simulink model "m02_PMSM_HDL"  (R2023b)
settings: Solver=FixedStepDiscrete  StartTime=0.0  StopTime=0.6  RelTol=1e-3  AbsTol=1e-3
PreLoadFcn:
  | control_data;
  | pmsm_data;
  | 
  | avgFactor = 1;
undefined symbols (not defined in the file): ee_sli_rtmsupport, f1478573793584, f1859323186544, fsw, gcbh, J, Ld, Lq, N, PM, Pmax, Tmax, Ts, Tsc
libraries: hdlssclib x24, simulink x8, SimscapeFPGAHIL_lib x6, fpga_utils_lib x5, hdlsllib x4, eeTransforms x2, eePwmGeneratorTwoLevel x1, eePmsmCurrentController x1, eePmsmCurrentReferenceGen x1, eeVelocityController x1
(part 3 of 3)

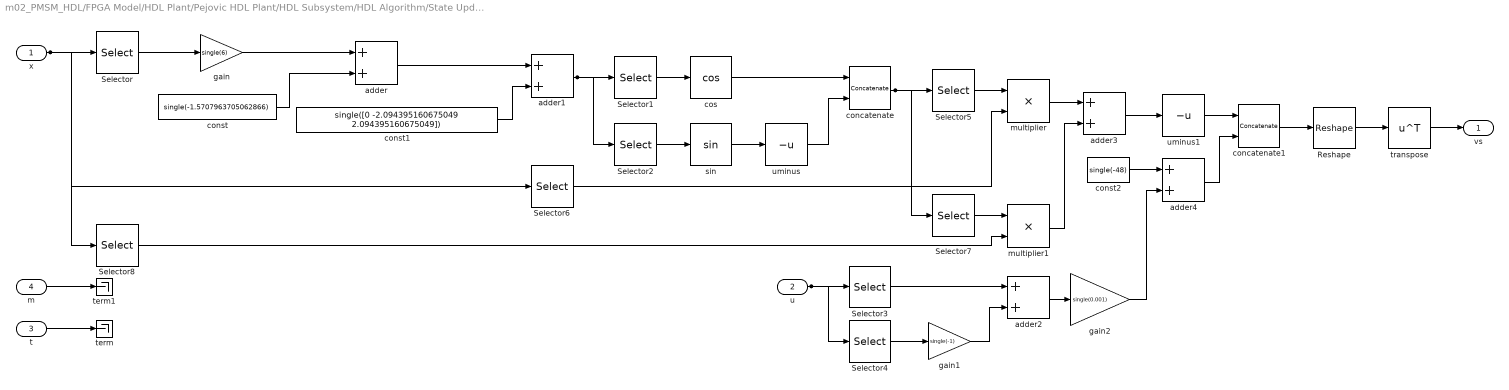
== system m02_PMSM_HDL/FPGA Model/HDL Plant/Pejovic HDL Plant/HDL Subsystem/HDL Algorithm/State Update/Algebraic Clump4/extClump3_F ==
  x : Inport  OutDataTypeStr=single  PortDimensions=[5 1]  SampleTime=2.5e-06
  u : Inport  Port=2  OutDataTypeStr=single  PortDimensions=[2 1]  SampleTime=2.5e-06
  t : Inport  Port=3  OutDataTypeStr=single  SampleTime=2.5e-06
  m : Inport  Port=4  OutDataTypeStr=int32  SampleTime=2.5e-06
  Reshape : Reshape  OutputDimensionality=Column vector (2-D)
  Selector : Selector  SampleTime=2.5e-06  IndexOptions=Index vector (dialog)  Indices=double(3)  OutputSizes=double(0)
  Selector{1..3,5} (4 alike) : Selector  SampleTime=2.5e-06  IndexOptions=Index vector (dialog)  Indices=double(1)  OutputSizes=double(0)
  Selector4 : Selector  SampleTime=2.5e-06  IndexOptions=Index vector (dialog)  Indices=double(2)  OutputSizes=double(0)
  Selector6 : Selector  SampleTime=2.5e-06  IndexOptions=Index vector (dialog)  Indices=double(4)  OutputSizes=double(0)
  Selector7 : Selector  SampleTime=2.5e-06  IndexOptions=Index vector (dialog)  Indices=double(2)  OutputSizes=double(0)
  Selector8 : Selector  SampleTime=2.5e-06  IndexOptions=Index vector (dialog)  Indices=double(5)  OutputSizes=double(0)
  adder{,1..4} (5 alike) : Sum  OutDataTypeStr=single  AccumDataTypeStr=single  SampleTime=2.5e-06
  concatenate : Concatenate  Mode=Multidimensional array  ConcatenateDimension=2
  concatenate1 : Concatenate  Mode=Multidimensional array
  const : Constant  Value=single(-1.5707963705062866)  VectorParams1D=off  OutDataTypeStr=single  SampleTime=2.5e-06
  const1 : Constant  Value=single([0 -2.094395160675049 2.094395160675049])  VectorParams1D=off  OutDataTypeStr=single  SampleTime=2.5e-06
  const2 : Constant  Value=single(-48)  VectorParams1D=off  OutDataTypeStr=single  SampleTime=2.5e-06
  cos : Trigonometry  Operator=cos  SampleTime=2.5e-06
  gain : Gain  Gain=single(6)  OutDataTypeStr=single  SampleTime=2.5e-06
  gain1 : Gain  Gain=single(-1)  OutDataTypeStr=single  SampleTime=2.5e-06
  gain2 : Gain  Gain=single(0.001)  OutDataTypeStr=single  SampleTime=2.5e-06
  multiplier : Product  Inputs=**  OutDataTypeStr=single  SampleTime=2.5e-06
  multiplier1 : Product  Inputs=**  OutDataTypeStr=single  SampleTime=2.5e-06
  sin : Trigonometry  SampleTime=2.5e-06
  term : Terminator
  term1 : Terminator
  transpose : Math  Operator=transpose
  uminus : UnaryMinus  SampleTime=2.5e-06
  uminus1 : UnaryMinus  SampleTime=2.5e-06
  vs : Outport  OutDataTypeStr=single  PortDimensions=[1 2]  SampleTime=2.5e-06
  wires:
  u/1 -> Selector4/1, Selector3/1
  x/1 -> Selector6/1, Selector8/1, Selector/1
  m/1 -> term1/1
  t/1 -> term/1
  Reshape/1 -> transpose/1
  Selector/1 -> gain/1
  Selector7/1 -> multiplier1/1
  Selector8/1 -> multiplier1/2
  cos/1 -> concatenate/1
  gain/1 -> adder/1
  const2/1 -> adder4/1
  const1/1 -> adder1/2
  const/1 -> adder/2
  adder/1 -> adder1/1
  adder2/1 -> gain2/1
  adder1/1 -> Selector2/1, Selector1/1
  Selector5/1 -> multiplier/1
  Selector6/1 -> multiplier/2
  Selector2/1 -> sin/1
  Selector1/1 -> cos/1
  multiplier1/1 -> adder3/2
  sin/1 -> uminus/1
  transpose/1 -> vs/1
  uminus/1 -> concatenate/2
  concatenate1/1 -> Reshape/1
  concatenate/1 -> Selector7/1, Selector5/1
  Selector4/1 -> gain1/1
  Selector3/1 -> adder2/1
  gain2/1 -> adder4/2
  gain1/1 -> adder2/2
  multiplier/1 -> adder3/1
  adder3/1 -> uminus1/1
  uminus1/1 -> concatenate1/1
  adder4/1 -> concatenate1/2

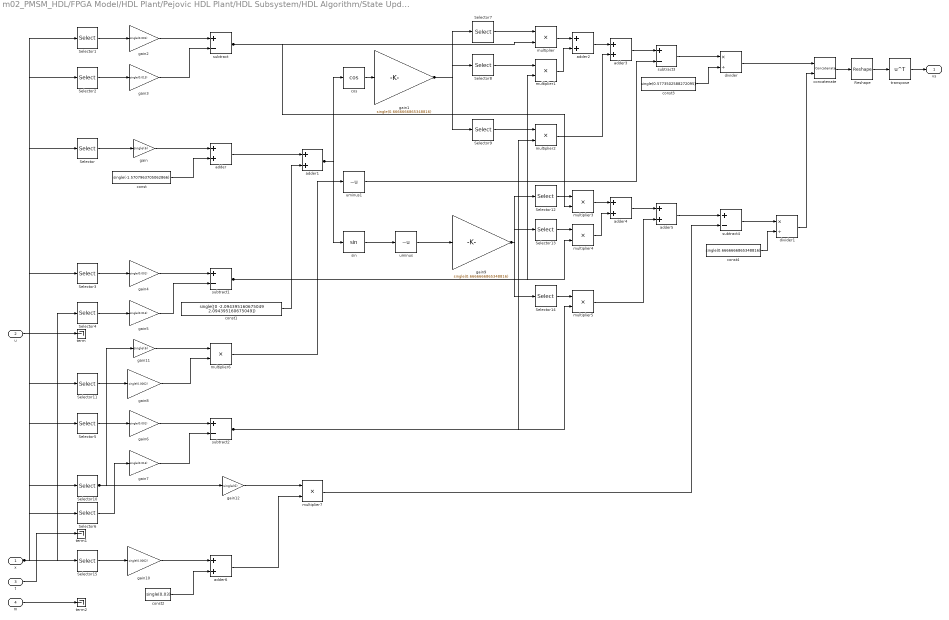
== system m02_PMSM_HDL/FPGA Model/HDL Plant/Pejovic HDL Plant/HDL Subsystem/HDL Algorithm/State Update/Differential Clump/diffClump_F ==
  x : Inport  OutDataTypeStr=single  PortDimensions=[12 1]  SampleTime=2.5e-06
  u : Inport  Port=2  OutDataTypeStr=single  PortDimensions=[6 1]  SampleTime=2.5e-06
  t : Inport  Port=3  OutDataTypeStr=single  SampleTime=2.5e-06
  m : Inport  Port=4  OutDataTypeStr=int32  SampleTime=2.5e-06
  Reshape : Reshape  OutputDimensionality=Column vector (2-D)
  Selector : Selector  SampleTime=2.5e-06  IndexOptions=Index vector (dialog)  Indices=double(10)  OutputSizes=double(0)
  Selector1 : Selector  SampleTime=2.5e-06  IndexOptions=Index vector (dialog)  Indices=double(1)  OutputSizes=double(0)
  Selector10 : Selector  SampleTime=2.5e-06  IndexOptions=Index vector (dialog)  Indices=double(7)  OutputSizes=double(0)
  Selector11 : Selector  SampleTime=2.5e-06  IndexOptions=Index vector (dialog)  Indices=double(12)  OutputSizes=double(0)
  Selector12 : Selector  SampleTime=2.5e-06  IndexOptions=Index vector (dialog)  Indices=double(1)  OutputSizes=double(0)
  Selector13 : Selector  SampleTime=2.5e-06  IndexOptions=Index vector (dialog)  Indices=double(2)  OutputSizes=double(0)
  Selector14 : Selector  SampleTime=2.5e-06  IndexOptions=Index vector (dialog)  Indices=double(3)  OutputSizes=double(0)
  Selector15 : Selector  SampleTime=2.5e-06  IndexOptions=Index vector (dialog)  Indices=double(11)  OutputSizes=double(0)
  Selector2 : Selector  SampleTime=2.5e-06  IndexOptions=Index vector (dialog)  Indices=double(4)  OutputSizes=double(0)
  Selector3 : Selector  SampleTime=2.5e-06  IndexOptions=Index vector (dialog)  Indices=double(2)  OutputSizes=double(0)
  Selector4 : Selector  SampleTime=2.5e-06  IndexOptions=Index vector (dialog)  Indices=double(5)  OutputSizes=double(0)
  Selector5 : Selector  SampleTime=2.5e-06  IndexOptions=Index vector (dialog)  Indices=double(3)  OutputSizes=double(0)
  Selector6 : Selector  SampleTime=2.5e-06  IndexOptions=Index vector (dialog)  Indices=double(6)  OutputSizes=double(0)
  Selector7 : Selector  SampleTime=2.5e-06  IndexOptions=Index vector (dialog)  Indices=double(1)  OutputSizes=double(0)
  Selector8 : Selector  SampleTime=2.5e-06  IndexOptions=Index vector (dialog)  Indices=double(2)  OutputSizes=double(0)
  Selector9 : Selector  SampleTime=2.5e-06  IndexOptions=Index vector (dialog)  Indices=double(3)  OutputSizes=double(0)
  adder{,1..6} (7 alike) : Sum  OutDataTypeStr=single  AccumDataTypeStr=single  SampleTime=2.5e-06
  concatenate : Concatenate  Mode=Multidimensional array
  const : Constant  Value=single(-1.5707963705062866)  VectorParams1D=off  OutDataTypeStr=single  SampleTime=2.5e-06
  const1 : Constant  Value=single([0 -2.094395160675049 2.094395160675049])  VectorParams1D=off  OutDataTypeStr=single  SampleTime=2.5e-06
  const2 : Constant  Value=single(0.03)  VectorParams1D=off  OutDataTypeStr=single  SampleTime=2.5e-06
  const3 : Constant  Value=single(0.5773502588272095)  VectorParams1D=off  OutDataTypeStr=single  SampleTime=2.5e-06
  const4 : Constant  Value=single(0.6666666865348816)  VectorParams1D=off  OutDataTypeStr=single  SampleTime=2.5e-06
  cos : Trigonometry  Operator=cos  SampleTime=2.5e-06
  divider : Product  Inputs=*/  OutDataTypeStr=single  SampleTime=2.5e-06
  divider1 : Product  Inputs=*/  OutDataTypeStr=single  SampleTime=2.5e-06
  gain : Gain  Gain=single(6)  OutDataTypeStr=single  SampleTime=2.5e-06
  gain1 : Gain  Gain=single(0.6666666865348816)  OutDataTypeStr=single  SampleTime=2.5e-06
  gain10 : Gain  Gain=single(0.0002)  OutDataTypeStr=single  SampleTime=2.5e-06
  gain11 : Gain  Gain=single(6)  OutDataTypeStr=single  SampleTime=2.5e-06
  gain12 : Gain  Gain=single(6)  OutDataTypeStr=single  SampleTime=2.5e-06
  gain2 : Gain  Gain=single(0.001)  OutDataTypeStr=single  SampleTime=2.5e-06
  gain3 : Gain  Gain=single(0.013)  OutDataTypeStr=single  SampleTime=2.5e-06
  gain4 : Gain  Gain=single(0.001)  OutDataTypeStr=single  SampleTime=2.5e-06
  gain5 : Gain  Gain=single(0.013)  OutDataTypeStr=single  SampleTime=2.5e-06
  gain6 : Gain  Gain=single(0.001)  OutDataTypeStr=single  SampleTime=2.5e-06
  gain7 : Gain  Gain=single(0.013)  OutDataTypeStr=single  SampleTime=2.5e-06
  gain8 : Gain  Gain=single(0.0002)  OutDataTypeStr=single  SampleTime=2.5e-06
  gain9 : Gain  Gain=single(0.6666666865348816)  OutDataTypeStr=single  SampleTime=2.5e-06
  multiplier{,1..7} (8 alike) : Product  Inputs=**  OutDataTypeStr=single  SampleTime=2.5e-06
  sin : Trigonometry  SampleTime=2.5e-06
  subtract{,1..4} (5 alike) : Sum  Inputs=+-  OutDataTypeStr=single  AccumDataTypeStr=single  SampleTime=2.5e-06
  term : Terminator
  term1 : Terminator
  term2 : Terminator
  transpose : Math  Operator=transpose
  uminus : UnaryMinus  SampleTime=2.5e-06
  uminus1 : UnaryMinus  SampleTime=2.5e-06
  vs : Outport  OutDataTypeStr=single  PortDimensions=[1 2]  SampleTime=2.5e-06
  wires:
  u/1 -> term/1
  t/1 -> term1/1
  adder5/1 -> subtract4/1
  x/1 -> Selector6/1, Selector3/1, Selector1/1, Selector4/1, Selector15/1, Selector2/1, Selector5/1, Selector/1, Selector11/1, Selector10/1
  m/1 -> term2/1
  Selector1/1 -> gain2/1
  Selector/1 -> gain/1
  Selector2/1 -> gain3/1
  Selector3/1 -> gain4/1
  gain3/1 -> subtract/2
  gain2/1 -> subtract/1
  Selector5/1 -> gain6/1
  Selector4/1 -> gain5/1
  Selector10/1 -> gain12/1, gain11/1
  divider/1 -> concatenate/1
  Selector11/1 -> gain8/1
  adder4/1 -> adder5/1
  Selector7/1 -> multiplier/1
  Selector6/1 -> gain7/1
  Selector14/1 -> multiplier5/1
  Selector15/1 -> gain10/1
  divider1/1 -> concatenate/2
  gain/1 -> adder/1
  const3/1 -> divider/2
  const1/1 -> adder1/2
  const2/1 -> adder6/2
  const/1 -> adder/2
  gain5/1 -> subtract1/2
  gain4/1 -> subtract1/1
  gain12/1 -> multiplier7/1
  gain11/1 -> multiplier6/1
  gain9/1 -> Selector14/1, Selector12/1, Selector13/1
  gain8/1 -> multiplier6/2
  gain7/1 -> subtract2/2
  gain6/1 -> subtract2/1
  gain1/1 -> Selector8/1, Selector7/1, Selector9/1
  gain10/1 -> adder6/1
  sin/1 -> uminus/1
  subtract/1 -> multiplier/2, multiplier3/2
  adder/1 -> adder1/1
  subtract1/1 -> multiplier4/2, multiplier1/2
  multiplier5/1 -> adder5/2
  multiplier6/1 -> uminus1/1
  subtract2/1 -> multiplier5/2, multiplier2/2
  adder6/1 -> multiplier7/2
  adder1/1 -> sin/1, cos/1
  multiplier7/1 -> subtract4/2
  const4/1 -> divider1/2
  cos/1 -> gain1/1
  uminus1/1 -> subtract3/2
  uminus/1 -> gain9/1
  Selector9/1 -> multiplier2/1
  Selector8/1 -> multiplier1/1
  multiplier/1 -> adder2/1
  multiplier2/1 -> adder3/2
  multiplier1/1 -> adder2/2
  Selector13/1 -> multiplier4/1
  Selector12/1 -> multiplier3/1
  adder3/1 -> subtract3/1
  adder2/1 -> adder3/1
  multiplier3/1 -> adder4/1
  multiplier4/1 -> adder4/2
  subtract4/1 -> divider1/1
  subtract3/1 -> divider/1
  concatenate/1 -> Reshape/1
  Reshape/1 -> transpose/1
  transpose/1 -> vs/1

== system m02_PMSM_HDL/FPGA Model/HDL Plant/Standard HDL Plant/HDL Subsystem/HDL Algorithm/State Update/Algebraic Clump1/extClump0_F ==
  x : Inport  OutDataTypeStr=single  PortDimensions=[6 1]  SampleTime=2.5e-06
  u : Inport  Port=2  OutDataTypeStr=single  SampleTime=2.5e-06
  t : Inport  Port=3  OutDataTypeStr=single  SampleTime=2.5e-06
  m : Inport  Port=4  OutDataTypeStr=int32  SampleTime=2.5e-06
  Reshape : Reshape  OutputDimensionality=Column vector (2-D)
  Selector : Selector  IndexOptions=Index vector (dialog)  Indices=double(5)  OutputSizes=double(0)
  Selector1 : Selector  IndexOptions=Index vector (dialog)  Indices=double(6)  OutputSizes=double(0)
  Selector2 : Selector  IndexOptions=Index vector (dialog)  Indices=double(6)  OutputSizes=double(0)
  Selector3 : Selector  IndexOptions=Index vector (dialog)  Indices=double(5)  OutputSizes=double(0)
  adder : Sum  OutDataTypeStr=single  AccumDataTypeStr=single  SampleTime=2.5e-06
  concatenate : Concatenate  NumInputs=4  Mode=Multidimensional array
  const : Constant  Value=single(0.03)  VectorParams1D=off  OutDataTypeStr=single  SampleTime=2.5e-06
  const1 : Constant  Value=single(0)  VectorParams1D=off  OutDataTypeStr=single  SampleTime=2.5e-06
  const2 : Constant  Value=single(0)  VectorParams1D=off  OutDataTypeStr=single  SampleTime=2.5e-06
  const3 : Constant  Value=single(0)  VectorParams1D=off  OutDataTypeStr=single  SampleTime=2.5e-06
  gain : Gain  Gain=single(0.0002)  OutDataTypeStr=single  SampleTime=2.5e-06
  gain1 : Gain  Gain=single(0.0002)  OutDataTypeStr=single  SampleTime=2.5e-06
  gain2 : Gain  Gain=single(9)  OutDataTypeStr=single  SampleTime=2.5e-06
  multiplier : Product  Inputs=**  OutDataTypeStr=single  SampleTime=2.5e-06
  multiplier1 : Product  Inputs=**  OutDataTypeStr=single  SampleTime=2.5e-06
  subtract : Sum  Inputs=+-  OutDataTypeStr=single  AccumDataTypeStr=single  SampleTime=2.5e-06
  term : Terminator
  term1 : Terminator
  term2 : Terminator
  transpose : Math  Operator=transpose
  uminus : UnaryMinus  SampleTime=2.5e-06
  vs : Outport  OutDataTypeStr=single  PortDimensions=[1 4]  SampleTime=2.5e-06
  wires:
  u/1 -> term/1
  x/1 -> Selector3/1, Selector2/1, Selector1/1, Selector/1
  t/1 -> term1/1
  m/1 -> term2/1
  const1/1 -> concatenate/2
  const/1 -> adder/2
  Selector/1 -> gain/1
  Selector1/1 -> gain1/1
  gain/1 -> adder/1
  Selector3/1 -> multiplier1/1
  gain1/1 -> multiplier1/2
  Selector2/1 -> multiplier/1
  adder/1 -> multiplier/2
  multiplier1/1 -> subtract/2
  multiplier/1 -> subtract/1
  transpose/1 -> vs/1
  subtract/1 -> gain2/1
  gain2/1 -> uminus/1
  uminus/1 -> concatenate/1
  const3/1 -> concatenate/4
  const2/1 -> concatenate/3
  concatenate/1 -> Reshape/1
  Reshape/1 -> transpose/1

== system m02_PMSM_HDL/FPGA Model/HDL Plant/Standard HDL Plant/HDL Subsystem/HDL Algorithm/State Update/Algebraic Clump2/Mode Vector To Index ==
  In1 : Inport
  State Mode Vector To Index : hdlssclib/HDL Logic Table  InputTable=[1 0;0 1]  OutputTable=[false;true]
  assertion : Assertion  StopWhenAssertionFail=off
  concat : hdlsllib/Logic and Bit Operations/Bit Concat  numInputs=1
  uncatalogued mode identifier : hdlssclib/HDL Logic Table  InputTable=[1 0;0 1]  OutputTable=[1;1]
  Out1 : Outport  VectorParamsAs1DForOutWhenUnconnected=off
  wires:
  State Mode Vector To Index/1 -> concat/1
  In1/1 -> State Mode Vector To Index/1, uncatalogued mode identifier/1
  uncatalogued mode identifier/1 -> assertion/1
  concat/1 -> Out1/1

== system m02_PMSM_HDL/FPGA Model/HDL Plant/Standard HDL Plant/HDL Subsystem/HDL Algorithm/State Update/Algebraic Clump2/Mode Vector Type Conversion ==
  Mode vec : Inport
  Data Type Conversion : DataTypeConversion  OutDataTypeStr=boolean  RndMeth=Nearest  SaturateOnIntegerOverflow=off
  Out1 : Outport  VectorParamsAs1DForOutWhenUnconnected=off
  wires:
  Mode vec/1 -> Data Type Conversion/1
  Data Type Conversion/1 -> Out1/1

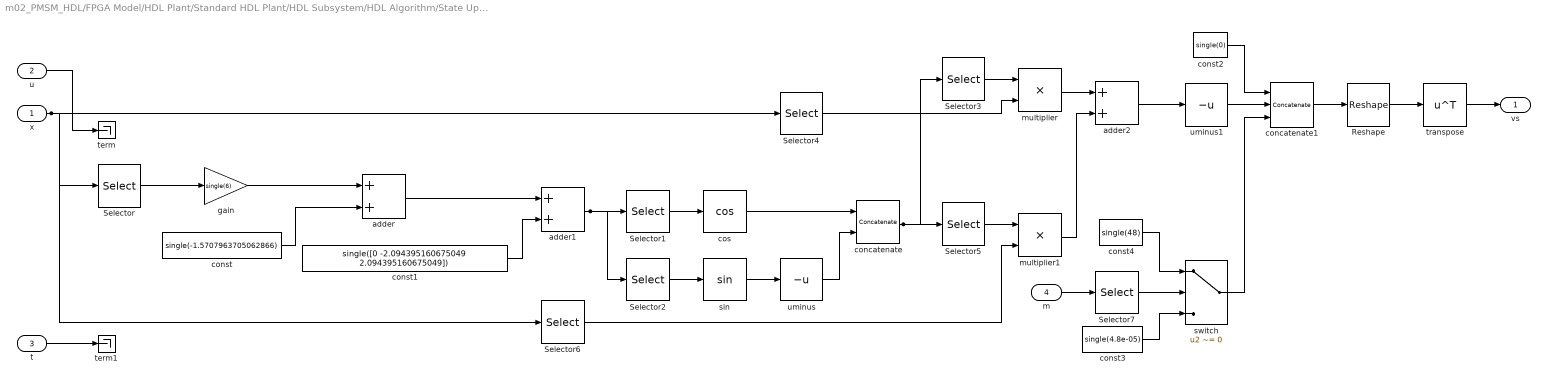
== system m02_PMSM_HDL/FPGA Model/HDL Plant/Standard HDL Plant/HDL Subsystem/HDL Algorithm/State Update/Algebraic Clump2/extClump1_F ==
  x : Inport  OutDataTypeStr=single  PortDimensions=[6 1]  SampleTime=2.5e-06
  u : Inport  Port=2  OutDataTypeStr=single  PortDimensions=[2 1]  SampleTime=2.5e-06
  t : Inport  Port=3  OutDataTypeStr=single  SampleTime=2.5e-06
  m : Inport  Port=4  OutDataTypeStr=int32  PortDimensions=[2 1]  SampleTime=2.5e-06
  Reshape : Reshape  OutputDimensionality=Column vector (2-D)
  Selector : Selector  IndexOptions=Index vector (dialog)  Indices=double(4)  OutputSizes=double(0)
  Selector1 : Selector  IndexOptions=Index vector (dialog)  Indices=double(3)  OutputSizes=double(0)
  Selector2 : Selector  IndexOptions=Index vector (dialog)  Indices=double(3)  OutputSizes=double(0)
  Selector3 : Selector  IndexOptions=Index vector (dialog)  Indices=double(1)  OutputSizes=double(0)
  Selector4 : Selector  IndexOptions=Index vector (dialog)  Indices=double(5)  OutputSizes=double(0)
  Selector5 : Selector  IndexOptions=Index vector (dialog)  Indices=double(2)  OutputSizes=double(0)
  Selector6 : Selector  IndexOptions=Index vector (dialog)  Indices=double(6)  OutputSizes=double(0)
  Selector7 : Selector  IndexOptions=Index vector (dialog)  Indices=double(1)  OutputSizes=double(0)
  adder : Sum  OutDataTypeStr=single  AccumDataTypeStr=single  SampleTime=2.5e-06
  adder1 : Sum  OutDataTypeStr=single  AccumDataTypeStr=single  SampleTime=2.5e-06
  adder2 : Sum  OutDataTypeStr=single  AccumDataTypeStr=single  SampleTime=2.5e-06
  concatenate : Concatenate  Mode=Multidimensional array  ConcatenateDimension=2
  concatenate1 : Concatenate  NumInputs=3  Mode=Multidimensional array
  const : Constant  Value=single(-1.5707963705062866)  VectorParams1D=off  OutDataTypeStr=single  SampleTime=2.5e-06
  const1 : Constant  Value=single([0 -2.094395160675049 2.094395160675049])  VectorParams1D=off  OutDataTypeStr=single  SampleTime=2.5e-06
  const2 : Constant  Value=single(0)  VectorParams1D=off  OutDataTypeStr=single  SampleTime=2.5e-06
  const3 : Constant  Value=single(4.8e-05)  VectorParams1D=off  OutDataTypeStr=single  SampleTime=2.5e-06
  const4 : Constant  Value=single(48)  VectorParams1D=off  OutDataTypeStr=single  SampleTime=2.5e-06
  cos : Trigonometry  Operator=cos  SampleTime=2.5e-06
  gain : Gain  Gain=single(6)  OutDataTypeStr=single  SampleTime=2.5e-06
  multiplier : Product  Inputs=**  OutDataTypeStr=single  SampleTime=2.5e-06
  multiplier1 : Product  Inputs=**  OutDataTypeStr=single  SampleTime=2.5e-06
  sin : Trigonometry  SampleTime=2.5e-06
  switch : Switch  Criteria=u2 ~= 0  Threshold=double(0)  OutDataTypeStr=single  SampleTime=2.5e-06  SaturateOnIntegerOverflow=off  InputSameDT=off
  term : Terminator
  term1 : Terminator
  transpose : Math  Operator=transpose
  uminus : UnaryMinus  SampleTime=2.5e-06
  uminus1 : UnaryMinus  SampleTime=2.5e-06
  vs : Outport  OutDataTypeStr=single  PortDimensions=[1 3]  SampleTime=2.5e-06
  wires:
  m/1 -> Selector7/1
  u/1 -> term/1
  x/1 -> Selector6/1, Selector/1, Selector4/1
  t/1 -> term1/1
  adder/1 -> adder1/1
  adder1/1 -> Selector2/1, Selector1/1
  Selector/1 -> gain/1
  multiplier1/1 -> adder2/2
  gain/1 -> adder/1
  const3/1 -> switch/3
  const1/1 -> adder1/2
  Reshape/1 -> transpose/1
  const2/1 -> concatenate1/1
  const4/1 -> switch/1
  cos/1 -> concatenate/1
  const/1 -> adder/2
  Selector7/1 -> switch/2
  Selector6/1 -> multiplier1/2
  Selector1/1 -> cos/1
  Selector2/1 -> sin/1
  transpose/1 -> vs/1
  switch/1 -> concatenate1/3
  sin/1 -> uminus/1
  Selector3/1 -> multiplier/1
  Selector4/1 -> multiplier/2
  uminus1/1 -> concatenate1/2
  uminus/1 -> concatenate/2
  concatenate1/1 -> Reshape/1
  concatenate/1 -> Selector5/1, Selector3/1
  Selector5/1 -> multiplier1/1
  multiplier/1 -> adder2/1
  adder2/1 -> uminus1/1

== system m02_PMSM_HDL/FPGA Model/HDL Plant/Standard HDL Plant/HDL Subsystem/HDL Algorithm/State Update/Algebraic Clump3/Mode Vector To Index ==
  In1 : Inport
  State Mode Vector To Index : hdlssclib/HDL Logic Table  InputTable=[1 0;0 1]  OutputTable=[false;true]
  assertion : Assertion  StopWhenAssertionFail=off
  concat : hdlsllib/Logic and Bit Operations/Bit Concat  numInputs=1
  uncatalogued mode identifier : hdlssclib/HDL Logic Table  InputTable=[1 0;0 1]  OutputTable=[1;1]
  Out1 : Outport  VectorParamsAs1DForOutWhenUnconnected=off
  wires:
  State Mode Vector To Index/1 -> concat/1
  In1/1 -> uncatalogued mode identifier/1, State Mode Vector To Index/1
  uncatalogued mode identifier/1 -> assertion/1
  concat/1 -> Out1/1

== system m02_PMSM_HDL/FPGA Model/HDL Plant/Standard HDL Plant/HDL Subsystem/HDL Algorithm/State Update/Algebraic Clump3/Mode Vector Type Conversion ==
  Mode vec : Inport
  Data Type Conversion : DataTypeConversion  OutDataTypeStr=boolean  RndMeth=Nearest  SaturateOnIntegerOverflow=off
  Out1 : Outport  VectorParamsAs1DForOutWhenUnconnected=off
  wires:
  Mode vec/1 -> Data Type Conversion/1
  Data Type Conversion/1 -> Out1/1

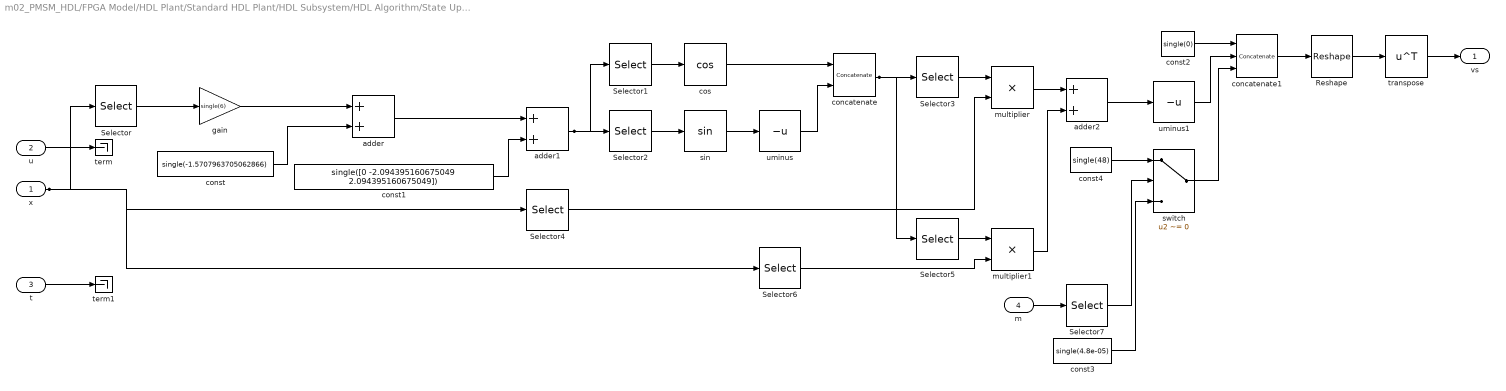
== system m02_PMSM_HDL/FPGA Model/HDL Plant/Standard HDL Plant/HDL Subsystem/HDL Algorithm/State Update/Algebraic Clump3/extClump2_F ==
  x : Inport  OutDataTypeStr=single  PortDimensions=[6 1]  SampleTime=2.5e-06
  u : Inport  Port=2  OutDataTypeStr=single  PortDimensions=[2 1]  SampleTime=2.5e-06
  t : Inport  Port=3  OutDataTypeStr=single  SampleTime=2.5e-06
  m : Inport  Port=4  OutDataTypeStr=int32  PortDimensions=[2 1]  SampleTime=2.5e-06
  Reshape : Reshape  OutputDimensionality=Column vector (2-D)
  Selector : Selector  IndexOptions=Index vector (dialog)  Indices=double(4)  OutputSizes=double(0)
  Selector1 : Selector  IndexOptions=Index vector (dialog)  Indices=double(2)  OutputSizes=double(0)
  Selector2 : Selector  IndexOptions=Index vector (dialog)  Indices=double(2)  OutputSizes=double(0)
  Selector3 : Selector  IndexOptions=Index vector (dialog)  Indices=double(1)  OutputSizes=double(0)
  Selector4 : Selector  IndexOptions=Index vector (dialog)  Indices=double(5)  OutputSizes=double(0)
  Selector5 : Selector  IndexOptions=Index vector (dialog)  Indices=double(2)  OutputSizes=double(0)
  Selector6 : Selector  IndexOptions=Index vector (dialog)  Indices=double(6)  OutputSizes=double(0)
  Selector7 : Selector  IndexOptions=Index vector (dialog)  Indices=double(1)  OutputSizes=double(0)
  adder : Sum  OutDataTypeStr=single  AccumDataTypeStr=single  SampleTime=2.5e-06
  adder1 : Sum  OutDataTypeStr=single  AccumDataTypeStr=single  SampleTime=2.5e-06
  adder2 : Sum  OutDataTypeStr=single  AccumDataTypeStr=single  SampleTime=2.5e-06
  concatenate : Concatenate  Mode=Multidimensional array  ConcatenateDimension=2
  concatenate1 : Concatenate  NumInputs=3  Mode=Multidimensional array
  const : Constant  Value=single(-1.5707963705062866)  VectorParams1D=off  OutDataTypeStr=single  SampleTime=2.5e-06
  const1 : Constant  Value=single([0 -2.094395160675049 2.094395160675049])  VectorParams1D=off  OutDataTypeStr=single  SampleTime=2.5e-06
  const2 : Constant  Value=single(0)  VectorParams1D=off  OutDataTypeStr=single  SampleTime=2.5e-06
  const3 : Constant  Value=single(4.8e-05)  VectorParams1D=off  OutDataTypeStr=single  SampleTime=2.5e-06
  const4 : Constant  Value=single(48)  VectorParams1D=off  OutDataTypeStr=single  SampleTime=2.5e-06
  cos : Trigonometry  Operator=cos  SampleTime=2.5e-06
  gain : Gain  Gain=single(6)  OutDataTypeStr=single  SampleTime=2.5e-06
  multiplier : Product  Inputs=**  OutDataTypeStr=single  SampleTime=2.5e-06
  multiplier1 : Product  Inputs=**  OutDataTypeStr=single  SampleTime=2.5e-06
  sin : Trigonometry  SampleTime=2.5e-06
  switch : Switch  Criteria=u2 ~= 0  Threshold=double(0)  OutDataTypeStr=single  SampleTime=2.5e-06  SaturateOnIntegerOverflow=off  InputSameDT=off
  term : Terminator
  term1 : Terminator
  transpose : Math  Operator=transpose
  uminus : UnaryMinus  SampleTime=2.5e-06
  uminus1 : UnaryMinus  SampleTime=2.5e-06
  vs : Outport  OutDataTypeStr=single  PortDimensions=[1 3]  SampleTime=2.5e-06
  wires:
  m/1 -> Selector7/1
  u/1 -> term/1
  t/1 -> term1/1
  x/1 -> Selector6/1, Selector4/1, Selector/1
  concatenate1/1 -> Reshape/1
  const/1 -> adder/2
  const1/1 -> adder1/2
  Reshape/1 -> transpose/1
  Selector/1 -> gain/1
  cos/1 -> concatenate/1
  gain/1 -> adder/1
  Selector7/1 -> switch/2
  adder/1 -> adder1/1
  adder1/1 -> Selector1/1, Selector2/1
  Selector3/1 -> multiplier/1
  Selector4/1 -> multiplier/2
  Selector2/1 -> sin/1
  Selector1/1 -> cos/1
  sin/1 -> uminus/1
  uminus1/1 -> concatenate1/2
  uminus/1 -> concatenate/2
  Selector5/1 -> multiplier1/1
  Selector6/1 -> multiplier1/2
  concatenate/1 -> Selector5/1, Selector3/1
  multiplier1/1 -> adder2/2
  multiplier/1 -> adder2/1
  adder2/1 -> uminus1/1
  const2/1 -> concatenate1/1
  const3/1 -> switch/3
  const4/1 -> switch/1
  transpose/1 -> vs/1
  switch/1 -> concatenate1/3

== system m02_PMSM_HDL/FPGA Model/HDL Plant/Standard HDL Plant/HDL Subsystem/HDL Algorithm/State Update/Algebraic Clump4/Mode Vector To Index ==
  In1 : Inport
  State Mode Vector To Index : hdlssclib/HDL Logic Table  InputTable=[1 0;0 1]  OutputTable=[false;true]
  assertion : Assertion  StopWhenAssertionFail=off
  concat : hdlsllib/Logic and Bit Operations/Bit Concat  numInputs=1
  uncatalogued mode identifier : hdlssclib/HDL Logic Table  InputTable=[1 0;0 1]  OutputTable=[1;1]
  Out1 : Outport  VectorParamsAs1DForOutWhenUnconnected=off
  wires:
  concat/1 -> Out1/1
  In1/1 -> State Mode Vector To Index/1, uncatalogued mode identifier/1
  uncatalogued mode identifier/1 -> assertion/1
  State Mode Vector To Index/1 -> concat/1

== system m02_PMSM_HDL/FPGA Model/HDL Plant/Standard HDL Plant/HDL Subsystem/HDL Algorithm/State Update/Algebraic Clump4/Mode Vector Type Conversion ==
  Mode vec : Inport
  Data Type Conversion : DataTypeConversion  OutDataTypeStr=boolean  RndMeth=Nearest  SaturateOnIntegerOverflow=off
  Out1 : Outport  VectorParamsAs1DForOutWhenUnconnected=off
  wires:
  Mode vec/1 -> Data Type Conversion/1
  Data Type Conversion/1 -> Out1/1

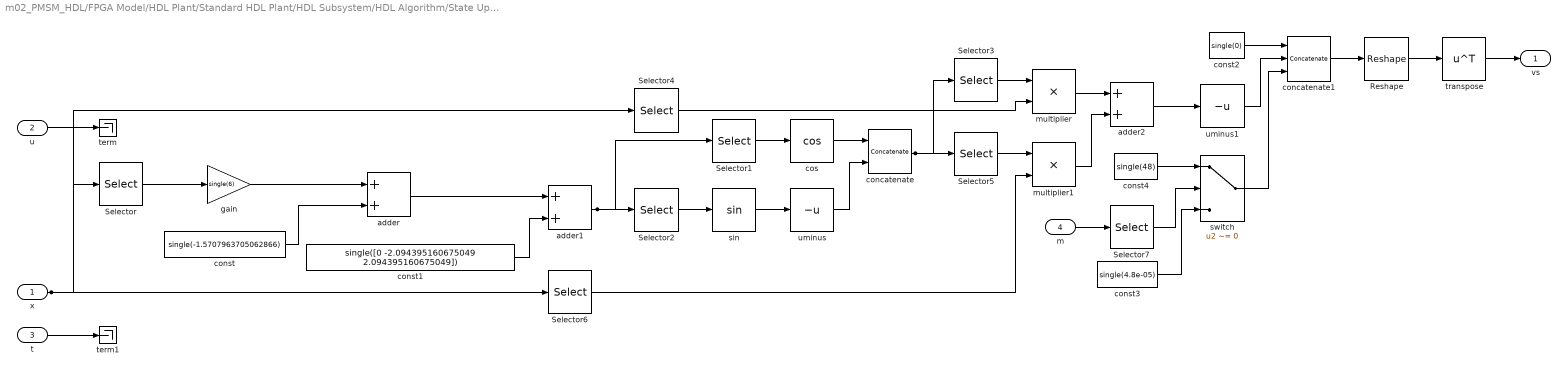
== system m02_PMSM_HDL/FPGA Model/HDL Plant/Standard HDL Plant/HDL Subsystem/HDL Algorithm/State Update/Algebraic Clump4/extClump3_F ==
  x : Inport  OutDataTypeStr=single  PortDimensions=[6 1]  SampleTime=2.5e-06
  u : Inport  Port=2  OutDataTypeStr=single  PortDimensions=[2 1]  SampleTime=2.5e-06
  t : Inport  Port=3  OutDataTypeStr=single  SampleTime=2.5e-06
  m : Inport  Port=4  OutDataTypeStr=int32  PortDimensions=[2 1]  SampleTime=2.5e-06
  Reshape : Reshape  OutputDimensionality=Column vector (2-D)
  Selector : Selector  IndexOptions=Index vector (dialog)  Indices=double(4)  OutputSizes=double(0)
  Selector{1..3,7} (4 alike) : Selector  IndexOptions=Index vector (dialog)  Indices=double(1)  OutputSizes=double(0)
  Selector4 : Selector  IndexOptions=Index vector (dialog)  Indices=double(5)  OutputSizes=double(0)
  Selector5 : Selector  IndexOptions=Index vector (dialog)  Indices=double(2)  OutputSizes=double(0)
  Selector6 : Selector  IndexOptions=Index vector (dialog)  Indices=double(6)  OutputSizes=double(0)
  adder : Sum  OutDataTypeStr=single  AccumDataTypeStr=single  SampleTime=2.5e-06
  adder1 : Sum  OutDataTypeStr=single  AccumDataTypeStr=single  SampleTime=2.5e-06
  adder2 : Sum  OutDataTypeStr=single  AccumDataTypeStr=single  SampleTime=2.5e-06
  concatenate : Concatenate  Mode=Multidimensional array  ConcatenateDimension=2
  concatenate1 : Concatenate  NumInputs=3  Mode=Multidimensional array
  const : Constant  Value=single(-1.5707963705062866)  VectorParams1D=off  OutDataTypeStr=single  SampleTime=2.5e-06
  const1 : Constant  Value=single([0 -2.094395160675049 2.094395160675049])  VectorParams1D=off  OutDataTypeStr=single  SampleTime=2.5e-06
  const2 : Constant  Value=single(0)  VectorParams1D=off  OutDataTypeStr=single  SampleTime=2.5e-06
  const3 : Constant  Value=single(4.8e-05)  VectorParams1D=off  OutDataTypeStr=single  SampleTime=2.5e-06
  const4 : Constant  Value=single(48)  VectorParams1D=off  OutDataTypeStr=single  SampleTime=2.5e-06
  cos : Trigonometry  Operator=cos  SampleTime=2.5e-06
  gain : Gain  Gain=single(6)  OutDataTypeStr=single  SampleTime=2.5e-06
  multiplier : Product  Inputs=**  OutDataTypeStr=single  SampleTime=2.5e-06
  multiplier1 : Product  Inputs=**  OutDataTypeStr=single  SampleTime=2.5e-06
  sin : Trigonometry  SampleTime=2.5e-06
  switch : Switch  Criteria=u2 ~= 0  Threshold=double(0)  OutDataTypeStr=single  SampleTime=2.5e-06  SaturateOnIntegerOverflow=off  InputSameDT=off
  term : Terminator
  term1 : Terminator
  transpose : Math  Operator=transpose
  uminus : UnaryMinus  SampleTime=2.5e-06
  uminus1 : UnaryMinus  SampleTime=2.5e-06
  vs : Outport  OutDataTypeStr=single  PortDimensions=[1 3]  SampleTime=2.5e-06
  wires:
  u/1 -> term/1
  x/1 -> Selector6/1, Selector4/1, Selector/1
  t/1 -> term1/1
  const2/1 -> concatenate1/1
  const3/1 -> switch/3
  const4/1 -> switch/1
  const1/1 -> adder1/2
  Selector1/1 -> cos/1
  Selector/1 -> gain/1
  cos/1 -> concatenate/1
  gain/1 -> adder/1
  concatenate1/1 -> Reshape/1
  const/1 -> adder/2
  adder/1 -> adder1/1
  adder2/1 -> uminus1/1
  adder1/1 -> Selector2/1, Selector1/1
  Selector7/1 -> switch/2
  Selector6/1 -> multiplier1/2
  Selector5/1 -> multiplier1/1
  Selector4/1 -> multiplier/2
  Selector3/1 -> multiplier/1
  Selector2/1 -> sin/1
  multiplier1/1 -> adder2/2
  sin/1 -> uminus/1
  transpose/1 -> vs/1
  uminus/1 -> concatenate/2
  concatenate/1 -> Selector5/1, Selector3/1
  multiplier/1 -> adder2/1
  Reshape/1 -> transpose/1
  m/1 -> Selector7/1
  uminus1/1 -> concatenate1/2
  switch/1 -> concatenate1/3

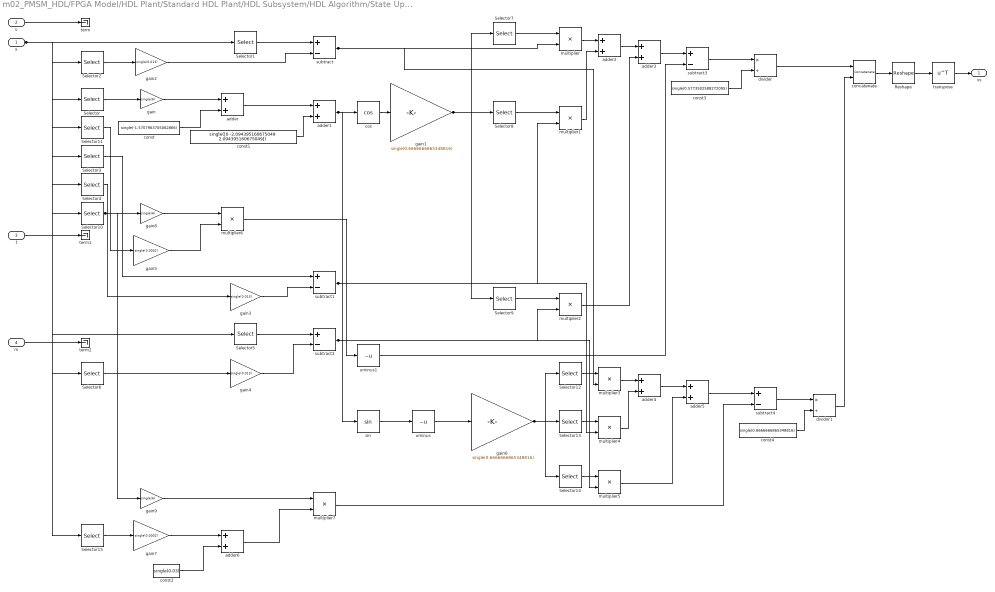
== system m02_PMSM_HDL/FPGA Model/HDL Plant/Standard HDL Plant/HDL Subsystem/HDL Algorithm/State Update/Differential Clump/diffClump_F ==
  x : Inport  OutDataTypeStr=single  PortDimensions=[15 1]  SampleTime=2.5e-06
  u : Inport  Port=2  OutDataTypeStr=single  PortDimensions=[6 1]  SampleTime=2.5e-06
  t : Inport  Port=3  OutDataTypeStr=single  SampleTime=2.5e-06
  m : Inport  Port=4  OutDataTypeStr=int32  PortDimensions=[6 1]  SampleTime=2.5e-06
  Reshape : Reshape  OutputDimensionality=Column vector (2-D)
  Selector : Selector  IndexOptions=Index vector (dialog)  Indices=double(13)  OutputSizes=double(0)
  Selector1 : Selector  IndexOptions=Index vector (dialog)  Indices=double(10)  OutputSizes=double(0)
  Selector10 : Selector  IndexOptions=Index vector (dialog)  Indices=double(7)  OutputSizes=double(0)
  Selector11 : Selector  IndexOptions=Index vector (dialog)  Indices=double(15)  OutputSizes=double(0)
  Selector12 : Selector  IndexOptions=Index vector (dialog)  Indices=double(1)  OutputSizes=double(0)
  Selector13 : Selector  IndexOptions=Index vector (dialog)  Indices=double(2)  OutputSizes=double(0)
  Selector14 : Selector  IndexOptions=Index vector (dialog)  Indices=double(3)  OutputSizes=double(0)
  Selector15 : Selector  IndexOptions=Index vector (dialog)  Indices=double(14)  OutputSizes=double(0)
  Selector2 : Selector  IndexOptions=Index vector (dialog)  Indices=double(4)  OutputSizes=double(0)
  Selector3 : Selector  IndexOptions=Index vector (dialog)  Indices=double(11)  OutputSizes=double(0)
  Selector4 : Selector  IndexOptions=Index vector (dialog)  Indices=double(5)  OutputSizes=double(0)
  Selector5 : Selector  IndexOptions=Index vector (dialog)  Indices=double(12)  OutputSizes=double(0)
  Selector6 : Selector  IndexOptions=Index vector (dialog)  Indices=double(6)  OutputSizes=double(0)
  Selector7 : Selector  IndexOptions=Index vector (dialog)  Indices=double(1)  OutputSizes=double(0)
  Selector8 : Selector  IndexOptions=Index vector (dialog)  Indices=double(2)  OutputSizes=double(0)
  Selector9 : Selector  IndexOptions=Index vector (dialog)  Indices=double(3)  OutputSizes=double(0)
  adder{,1..6} (7 alike) : Sum  OutDataTypeStr=single  AccumDataTypeStr=single  SampleTime=2.5e-06
  concatenate : Concatenate  Mode=Multidimensional array
  const : Constant  Value=single(-1.5707963705062866)  VectorParams1D=off  OutDataTypeStr=single  SampleTime=2.5e-06
  const1 : Constant  Value=single([0 -2.094395160675049 2.094395160675049])  VectorParams1D=off  OutDataTypeStr=single  SampleTime=2.5e-06
  const2 : Constant  Value=single(0.03)  VectorParams1D=off  OutDataTypeStr=single  SampleTime=2.5e-06
  const3 : Constant  Value=single(0.5773502588272095)  VectorParams1D=off  OutDataTypeStr=single  SampleTime=2.5e-06
  const4 : Constant  Value=single(0.6666666865348816)  VectorParams1D=off  OutDataTypeStr=single  SampleTime=2.5e-06
  cos : Trigonometry  Operator=cos  SampleTime=2.5e-06
  divider : Product  Inputs=*/  OutDataTypeStr=single  SampleTime=2.5e-06
  divider1 : Product  Inputs=*/  OutDataTypeStr=single  SampleTime=2.5e-06
  gain : Gain  Gain=single(6)  OutDataTypeStr=single  SampleTime=2.5e-06
  gain1 : Gain  Gain=single(0.6666666865348816)  OutDataTypeStr=single  SampleTime=2.5e-06
  gain2 : Gain  Gain=single(0.013)  OutDataTypeStr=single  SampleTime=2.5e-06
  gain3 : Gain  Gain=single(0.013)  OutDataTypeStr=single  SampleTime=2.5e-06
  gain4 : Gain  Gain=single(0.013)  OutDataTypeStr=single  SampleTime=2.5e-06
  gain5 : Gain  Gain=single(0.0002)  OutDataTypeStr=single  SampleTime=2.5e-06
  gain6 : Gain  Gain=single(0.6666666865348816)  OutDataTypeStr=single  SampleTime=2.5e-06
  gain7 : Gain  Gain=single(0.0002)  OutDataTypeStr=single  SampleTime=2.5e-06
  gain8 : Gain  Gain=single(6)  OutDataTypeStr=single  SampleTime=2.5e-06
  gain9 : Gain  Gain=single(6)  OutDataTypeStr=single  SampleTime=2.5e-06
  multiplier{,1..7} (8 alike) : Product  Inputs=**  OutDataTypeStr=single  SampleTime=2.5e-06
  sin : Trigonometry  SampleTime=2.5e-06
  subtract{,1..4} (5 alike) : Sum  Inputs=+-  OutDataTypeStr=single  AccumDataTypeStr=single  SampleTime=2.5e-06
  term : Terminator
  term1 : Terminator
  term2 : Terminator
  transpose : Math  Operator=transpose
  uminus : UnaryMinus  SampleTime=2.5e-06
  uminus1 : UnaryMinus  SampleTime=2.5e-06
  vs : Outport  OutDataTypeStr=single  PortDimensions=[1 2]  SampleTime=2.5e-06
  wires:
  uminus1/1 -> subtract3/2
  Selector11/1 -> gain5/1
  concatenate/1 -> Reshape/1
  x/1 -> Selector1/1, Selector5/1, Selector6/1, Selector4/1, Selector3/1, Selector10/1, Selector/1, Selector11/1, Selector15/1, Selector2/1
  u/1 -> term/1
  t/1 -> term1/1
  m/1 -> term2/1
  subtract4/1 -> divider1/1
  Selector/1 -> gain/1
  Selector2/1 -> gain2/1
  Selector3/1 -> subtract1/1
  Selector4/1 -> gain3/1
  uminus/1 -> gain6/1
  Selector10/1 -> gain9/1, gain8/1
  Selector6/1 -> gain4/1
  Selector15/1 -> gain7/1
  gain2/1 -> subtract/2
  gain/1 -> adder/1
  const1/1 -> adder1/2
  const/1 -> adder/2
  gain8/1 -> multiplier6/1
  gain5/1 -> multiplier6/2
  gain9/1 -> multiplier7/1
  gain7/1 -> adder6/1
  const3/1 -> divider/2
  const2/1 -> adder6/2
  transpose/1 -> vs/1
  Selector1/1 -> subtract/1
  adder/1 -> adder1/1
  multiplier6/1 -> uminus1/1
  gain3/1 -> subtract1/2
  Selector5/1 -> subtract2/1
  gain4/1 -> subtract2/2
  adder6/1 -> multiplier7/2
  subtract/1 -> multiplier3/2, multiplier/2
  adder1/1 -> sin/1, cos/1
  subtract1/1 -> multiplier4/2, multiplier1/2
  subtract2/1 -> multiplier5/2, multiplier2/2
  multiplier7/1 -> subtract4/2
  cos/1 -> gain1/1
  sin/1 -> uminus/1
  gain1/1 -> Selector9/1, Selector8/1, Selector7/1
  Selector7/1 -> multiplier/1
  Selector8/1 -> multiplier1/1
  Selector9/1 -> multiplier2/1
  gain6/1 -> Selector14/1, Selector13/1, Selector12/1
  multiplier/1 -> adder2/1
  multiplier1/1 -> adder2/2
  multiplier2/1 -> adder3/2
  Selector12/1 -> multiplier3/1
  Selector13/1 -> multiplier4/1
  Selector14/1 -> multiplier5/1
  adder2/1 -> adder3/1
  multiplier3/1 -> adder4/1
  multiplier4/1 -> adder4/2
  multiplier5/1 -> adder5/2
  adder3/1 -> subtract3/1
  adder4/1 -> adder5/1
  Reshape/1 -> transpose/1
  subtract3/1 -> divider/1
  adder5/1 -> subtract4/1
  divider/1 -> concatenate/1
  const4/1 -> divider1/2
  divider1/1 -> concatenate/2

== matlab function m02_PMSM_HDL/PMSM controller/PMSM Field-Oriented Control/PWM/PWM Generator (Three-phase, Two-level)/Switching Time Calculation ==
  settings: sampleTime=1
  data: Vabc input; TgabcON output; vdc input; TgabcOFF output; ModWave output; fsw parameter; PWM parameter
function [TgabcON,TgabcOFF,ModWave]  = switchingTime(Vabc,vdc,fsw,PWM)

[TgabcON,TgabcOFF,ModWave] = ee.control.pwmSwitchingTimeTwoLevel(Vabc,vdc,fsw,PWM);
